simulink model "arduino_send_serial"  (R2014a)
settings: Solver=ode3  SolverMode=SingleTasking  StartTime=0.0  StopTime=10.0  FixedStep=0.01  RelTol=1e-3
libraries: arduinolib x4
settings Model: ExtModeTrigDuration=2  Creator=Ulysses  LastModifiedBy=Ulysses
settings OptimizationCC: OptimizeModelRefInitCode=on  LifeSpan=1
settings DebuggingCC: UnderspecifiedInitializationDetection=Classic  SolverPrmCheckMsg=none
settings HardwareCC: ProdBitPerInt=16  ProdBitPerPointer=8  ProdIntDivRoundTo=Zero  ProdEndianess=LittleEndian  ProdWordSize=8  ProdHWDeviceType=Atmel->AVR
settings RTWCC: SystemTargetFile=realtime.tlc  GenerateMakefile=off  TemplateMakefile=realtime.tmf  Description=Run on Target Hardware  RTWVerbose=off  ProcessScript=realtime_make_rtw_hook
settings STFCustomTargetCC: TargetLibSuffix=.a  GenerateSampleERTMain=on  ConcurrentExecutionCompliant=off  GeneratePreprocessorConditionals=Use local settings  ERTCustomFileBanners=on  SupportNonInlinedSFcns=off  SupportVariableSizeSignals=on  MATLABClassNameForMDSCustomization=Simulink.SoftwareTarget.ERTCustomization  GRTInterface=off  SystemTargetFile=realtime.tlc
settings ERTTargetCC: CombineOutputUpdateFcns=off  SupportContinuousTime=on  SupportVariableSizeSignals=on  ExtModeTransport=3  ExtModeMexFile=ext_serial_win32_comm  ExtModeMexArgs=0 1 9600  ERTSrcFileBannerTemplate=realtime_code_template.cgt  ERTHdrFileBannerTemplate=realtime_code_template.cgt  ERTDataSrcFileTemplate=realtime_code_template.cgt  ERTDataHdrFileTemplate=realtime_code_template.cgt  ERTCustomFileTemplate=realtime_file_process.tlc

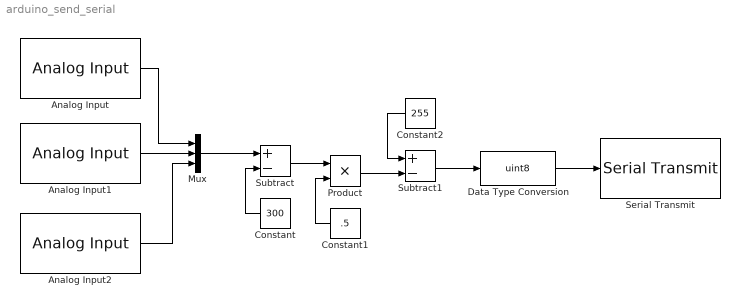
== system arduino_send_serial ==
  Analog Input : arduinolib/Analog Input  pinNumber=0  sampleTime=0.1
  Analog Input1 : arduinolib/Analog Input  pinNumber=1  sampleTime=0.1
  Analog Input2 : arduinolib/Analog Input  pinNumber=2  sampleTime=0.1
  Constant : Constant  Value=300
  Constant1 : Constant  Value=.5
  Constant2 : Constant  Value=255
  Data Type Conversion : DataTypeConversion  OutDataTypeStr=uint8  ConvertRealWorld=Stored Integer (SI)  RndMeth=Nearest
  Mux : Mux  Inputs=3
  Product : Product
  Serial Transmit : arduinolib/Serial Transmit  portNumber=0
  Subtract : Sum  Inputs=+-
  Subtract1 : Sum  Inputs=+-
  wires:
  Data Type Conversion/1 -> Serial Transmit/1
  Analog Input1/1 -> Mux/2
  Mux/1 -> Subtract/1
  Analog Input2/1 -> Mux/3
  Analog Input/1 -> Mux/1
  Constant/1 -> Subtract/2
  Subtract/1 -> Product/1
  Constant1/1 -> Product/2
  Constant2/1 -> Subtract1/1
  Product/1 -> Subtract1/2
  Subtract1/1 -> Data Type Conversion/1
